simulink model "desiredTaskSpacePassivityBasedController"  (R2024a)
settings: Solver=ode1  StartTime=0.0  StopTime=10  FixedStep=0.01  RelTol=1e-3
libraries: robotmaniplib x2, slpidlib x1
settings Model: Creator=gujun  LastModifiedBy=jun
settings RTWCC: GPUComputeCapability=3.5

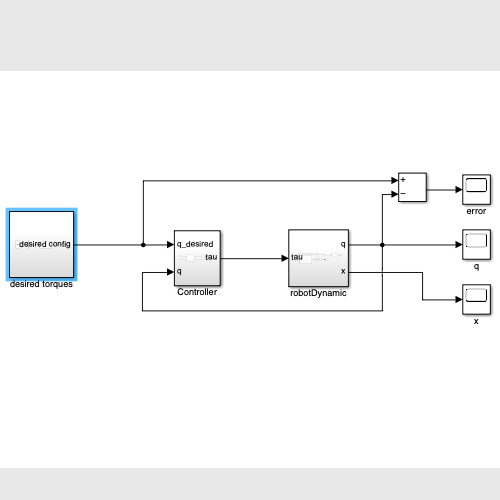
[thumbnail: Simulink's stored preview of the top-level diagram]
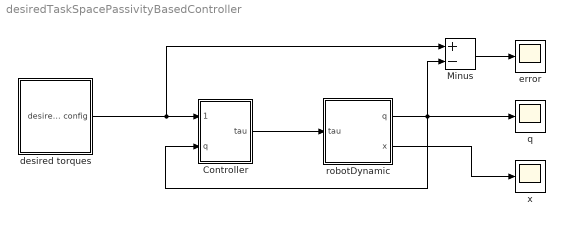
== system desiredTaskSpacePassivityBasedController ==
  Controller : Subsystem
  Minus : Sum  Inputs=+-
  desired torques : Subsystem
  error : Scope
  q : Scope
  robotDynamic : Subsystem
  x : Scope
  wires:
  robotDynamic/1(q) -> Controller/2(q), q/1, Minus/2
  desired torques/1(desired config) -> Minus/1, Controller/1(q_desired)
  Controller/1(tau) -> robotDynamic/1(tau)
  Minus/1 -> error/1
  robotDynamic/2(x) -> x/1

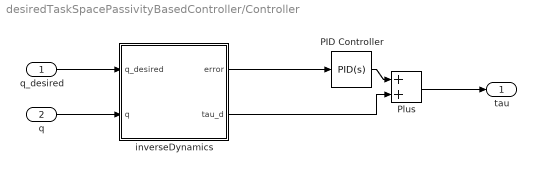
== system desiredTaskSpacePassivityBasedController/Controller ==
  q_desired : Inport
  q : Inport  Port=2
  PID Controller : slpidlib/PID Controller  Controller=PID  Form=Parallel  TimeDomain=Continuous-time  UseExternalTs=off  SampleTime=-1  IntegratorMethod=Forward Euler  FilterMethod=Forward Euler  ControllerParametersSource=internal  P=140  I=1  UseKiTs=off  D=20  UseExternalDerivativeSource=off  N=100  UseFilter=on  TunerSelectOption=Transfer Function Based (PID Tuner App)  InitialConditionSource=internal  InitialConditionForIntegrator=0  InitialConditionForFilter=0  DifferentiatorICPrevScaledInput=0  ExternalReset=none  TrackingMode=off  Kt=1  LimitOutput=off  SatLimitsSource=internal  UpperSaturationLimit=inf  LowerSaturationLimit=-inf  LinearizeAsGain=on  AntiWindupMode=none  Kb=1  LimitIntegrator=off  UpperIntegratorSaturationLimit=inf  LowerIntegratorSaturationLimit=-inf  POutMin=[]  POutMax=[]  IOutMin=[]  IOutMax=[]  DOutMin=[]  DOutMax=[]  NOutMin=[]  NOutMax=[]  SumOutMin=[]  SumOutMax=[]  SaturationOutMin=[]  SaturationOutMax=[]  PParamMin=[]  PParamMax=[]  IParamMin=[]  IParamMax=[]  DParamMin=[]  DParamMax=[]  NParamMin=[]  NParamMax=[]  KbParamMin=[]  KbParamMax=[]  KtParamMin=[]  KtParamMax=[]  KbOutMin=[]  KbOutMax=[]  KtOutMin=[]  KtOutMax=[]  IntegratorOutMin=[]  IntegratorOutMax=[]  FilterOutMin=[]  FilterOutMax=[]  SumI1OutMin=[]  SumI1OutMax=[]  SumI2OutMin=[]  SumI2OutMax=[]  SumI3OutMin=[]  SumI3OutMax=[]  SumI4OutMin=[]  SumI4OutMax=[]  SumDOutMin=[]  SumDOutMax=[]  DifferentiatorOutMin=[]  DifferentiatorOutMax=[]  FilterDiffOutCoefMin=[]  FilterDiffOutCoefMax=[]  ReciprocalOutMin=[]  ReciprocalOutMax=[]  SumDenOutMin=[]  SumDenOutMax=[]  SumNumOutMin=[]  SumNumOutMax=[]  DivideOutMin=[]  DivideOutMax=[]  UdiffTsProdOutMin=[]  UdiffTsProdOutMax=[]  NTsProdOutMin=[]  NTsProdOutMax=[]  UintegralTsProdOutMin=[]  UintegralTsProdOutMax=[]  UngainTsProdOutMin=[]  UngainTsProdOutMax=[]  ClampingZeroOutDataTypeStr=Inherit: Inherit via back propagation  ClampingZeroOutMin=[]  ClampingZeroOutMax=[]  FilterDenConstantOutDataTypeStr=Inherit: Inherit via back propagation  FilterDenConstantOutMin=[]  FilterDenConstantOutMax=[]  PCopyOutDataTypeStr=Inherit: Inherit via back propagation  PCopyOutMin=[]  PCopyOutMax=[]  NCopyOutDataTypeStr=Inherit: Inherit via back propagation  NCopyOutMin=[]  NCopyOutMax=[]  IntegratorContinuousStateAttributes=''  IntegratorStateMustResolveToSignalObject=off  IntegratorRTWStateStorageClass=Auto  FilterContinuousStateAttributes=''  FilterStateMustResolveToSignalObject=off  FilterRTWStateStorageClass=Auto  ParallelPVariant=InternalParameters  IdealPVariant=Disabled  IVariant=InternalParameters  DVariant=InternalParameters  IntegratorVariant=Continuous  SatVariant=Disabled  AWVariant=Passthrough  PCopyVariant=Disabled  TRVariant=Disabled  FdbkBlocksVariant=Forward  IdealPFdbkVariant=Disabled  SatFdbkVariant=Disabled  DerivativeFilterVariant=ContFilter  NVariant=InternalParameters  NCopyVariant=Disabled  FilterICVariant=InternalICsFilter  IntegratorICVariant=InternalICs  ExternalResetVariant=Disabled  TRSumVariant=Passthrough  SumFdbkVariant=Disabled  SumVariant=Sum_PID  TsampFilterVariant=InternalTs  TsampNgainVariant=Passthrough  TsampIntegralVariant=Disabled_SignalSpec  ExternalSaturationOutDataTypeStr=Inherit: Same as second input  DerivativeSourceVariant=ErrorSignal
  Plus : Sum
  inverseDynamics : Subsystem
  tau : Outport
  wires:
  q_desired/1 -> inverseDynamics/1(q_desired)
  inverseDynamics/2(tau_d) -> Plus/2
  Plus/1 -> tau/1
  q/1 -> inverseDynamics/2(q)
  inverseDynamics/1(error) -> PID Controller/1
  PID Controller/1 -> Plus/1

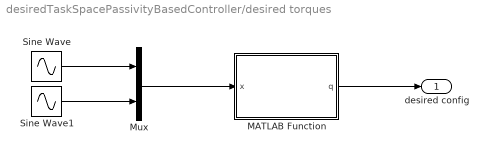
== system desiredTaskSpacePassivityBasedController/desired torques ==
  MATLAB Function : MATLAB Function  TreatAsAtomicUnit=on
  Mux : Mux  Inputs=2
  Sine Wave : Sin  Amplitude=0.2  SampleTime=0
  Sine Wave1 : Sin  Amplitude=0.2  Phase=pi/2  SampleTime=0
  desired config : Outport
  wires:
  Sine Wave1/1 -> Mux/2
  Sine Wave/1 -> Mux/1
  Mux/1 -> MATLAB Function/1(x)
  MATLAB Function/1(q) -> desired config/1

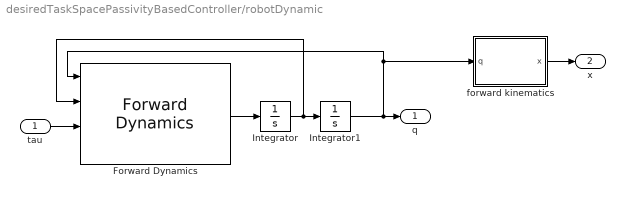
== system desiredTaskSpacePassivityBasedController/robotDynamic ==
  tau : Inport
  Forward Dynamics : robotmaniplib/Forward Dynamics  RigidBodyTree=twoJointSimpleRobot  SimulateUsing=Interpreted execution
  Integrator : Integrator
  Integrator1 : Integrator
  forward kinematics : MATLAB Function  TreatAsAtomicUnit=on
  q : Outport
  x : Outport  Port=2
  wires:
  Forward Dynamics/1 -> Integrator/1
  Integrator1/1 -> Forward Dynamics/1, forward kinematics/1(q), q/1
  Integrator/1 -> Forward Dynamics/2, Integrator1/1
  forward kinematics/1(x) -> x/1
  tau/1 -> Forward Dynamics/3

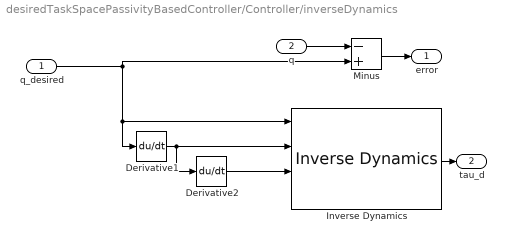
== system desiredTaskSpacePassivityBasedController/Controller/inverseDynamics ==
  q_desired : Inport
  q : Inport  Port=2
  Derivative1 : Derivative
  Derivative2 : Derivative
  Inverse Dynamics : robotmaniplib/Inverse Dynamics  RigidBodyTree=twoJointSimpleRobot  SimulateUsing=Interpreted execution
  Minus : Sum  Inputs=-+
  error : Outport
  tau_d : Outport  Port=2
  wires:
  q/1 -> Minus/1
  Derivative1/1 -> Inverse Dynamics/2, Derivative2/1
  q_desired/1 -> Minus/2, Inverse Dynamics/1, Derivative1/1
  Derivative2/1 -> Inverse Dynamics/3
  Minus/1 -> error/1
  Inverse Dynamics/1 -> tau_d/1

== matlab function desiredTaskSpacePassivityBasedController/robotDynamic/forward kinematics ==
  data: q input; x output
function x = kinematics(q)

lg1 = 0.2;
lg2 = 0.2;
x = [0;
    0];
x(1) = lg1 * cos(q(1)) + lg2 * cos(q(1) + q(2));
x(2) = lg1 * sin(q(1)) + lg2 * sin(q(1) + q(2));

end

== matlab function desiredTaskSpacePassivityBasedController/desired torques/MATLAB Function ==
  data: x input; q output
function q = ik(x)
    L1 = 0.2;
    L2 = 0.2;


    d = sqrt(x(1)^2 + x(2)^2);
    
    % Check if the point is reachable
    if d > (L1 + L2) || d < abs(L1 - L2)
        error('The point is not reachable.');
    end
    
    % Compute theta2 using the cosine law
    cosTheta2 = (x(1)^2 + x(2)^2 - L1^2 - L2^2) / (2 * L1 * L2);
    theta2 = acos(cosTheta2);
    
    % Compute the alternative theta2 (elbow down configuration)
    theta2_alt = -acos(cosTheta2);
    
    % Compute the intermediate values for theta1 calculation
    k1 = L1 + L2 * cos(theta2);
    k2 = L2 * sin(theta2);
    
    % Compute theta1
    theta1 = atan2(x(2), x(1)) - atan2(k2, k1);    
    
    % Compute the intermediate values for the alternative theta1
    k1_alt = L1 + L2 * cos(theta2_alt);
    k2_alt = L2 * sin(theta2_alt);
    


    q = [0; 0;];
    % Return the primary solution by default
    q(1) = theta1;
    q(2) = theta2;
end
